simulink model "Add_1simulink"  (R2022a)
settings: Solver=FixedStepAuto  StartTime=0.0  StopTime=3  FixedStep=0.0001  RelTol=1e-3
values from neighbouring files (symbols this model uses):
  J_motor = 0.000610871894223    [var_10.mat]
  L_phase = 0.00332259990587    [var_10.mat]
  M_nom = 0.61236365542    [var_10.mat]
  psi = 0.0961787034043    [var_10.mat]
  R_phase = 0.753894801324    [var_10.mat]
  U_nom = 48    [var_10.mat]
undefined symbols (not defined in the file or in its folder): Ki_i, Ki_w, Kp_i, Kp_w
libraries: simulink x1
settings Model: Creator=Family  LastModifiedBy=Family

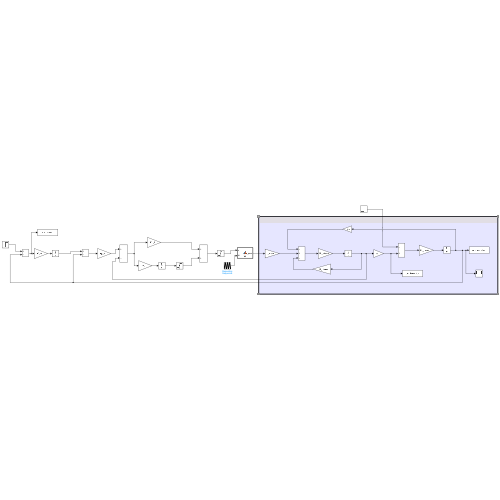
[thumbnail: Simulink's stored preview of the top-level diagram]
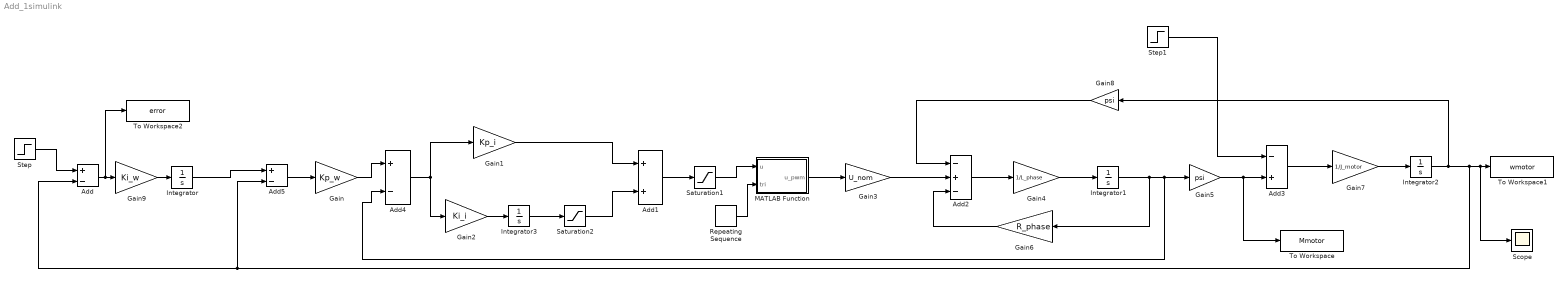
== system Add_1simulink ==
  Add : Sum  Inputs=+-
  Add1 : Sum
  Add2 : Sum  Inputs=-+-
  Add3 : Sum  Inputs=-+
  Add4 : Sum  Inputs=+-
  Add5 : Sum  Inputs=+-
  Gain : Gain  Gain=Kp_w
  Gain1 : Gain  Gain=Kp_i
  Gain2 : Gain  Gain=Ki_i
  Gain3 : Gain  Gain=U_nom
  Gain4 : Gain  Gain=1/L_phase
  Gain5 : Gain  Gain=psi
  Gain6 : Gain  Gain=R_phase
  Gain7 : Gain  Gain=1/J_motor
  Gain8 : Gain  Gain=psi
  Gain9 : Gain  Gain=Ki_w
  Integrator{,1..3} (4 alike) : Integrator
  MATLAB Function : MATLAB Function  TreatAsAtomicUnit=on
  Repeating Sequence : simulink/Sources/Repeating Sequence  rep_seq_t=[0 1/10000 1/5000]  rep_seq_y=[-1 1 -1]
  Saturation1 : Saturate  UpperLimit=1  LowerLimit=-1
  Saturation2 : Saturate  UpperLimit=1  LowerLimit=-1
  Scope : Scope
  Step : Step  Time=0.5  After=50  SampleTime=0
  Step1 : Step  Time=0.5  After=M_nom  SampleTime=0
  To Workspace : ToWorkspace  VariableName=Mmotor  SaveFormat=Timeseries  SampleTime=0.001
  To Workspace1 : ToWorkspace  VariableName=wmotor  SaveFormat=Timeseries  SampleTime=0.001
  To Workspace2 : ToWorkspace  VariableName=error  SaveFormat=Timeseries  SampleTime=0.001
  wires:
  Gain1/1 -> Add1/1
  Add1/1 -> Saturation1/1
  Gain2/1 -> Integrator3/1
  Add3/1 -> Gain7/1
  Integrator2/1 -> Add5/2, Add/2, Scope/1, To Workspace1/1, Gain8/1
  Gain7/1 -> Integrator2/1
  Gain6/1 -> Add2/3
  Gain5/1 -> To Workspace/1, Add3/2
  Gain4/1 -> Integrator1/1
  Add2/1 -> Gain4/1
  Gain3/1 -> Add2/2
  Integrator1/1 -> Gain6/1, Add4/2, Gain5/1
  Gain8/1 -> Add2/1
  Saturation1/1 -> MATLAB Function/1(u)
  Integrator3/1 -> Saturation2/1
  Saturation2/1 -> Add1/2
  Add4/1 -> Gain2/1, Gain1/1
  Gain/1 -> Add4/1
  Add/1 -> To Workspace2/1, Gain9/1
  Step/1 -> Add/1
  Gain9/1 -> Integrator/1
  Integrator/1 -> Add5/1
  MATLAB Function/1(u_pwm) -> Gain3/1
  Repeating Sequence/1 -> MATLAB Function/2(tri)
  Step1/1 -> Add3/1
  Add5/1 -> Gain/1

== matlab function Add_1simulink/MATLAB Function ==
  data: u input; u_pwm output; tri input
function u_pwm = fcn(u,tri)
if u >= tri
    u_pwm = 1;
else
    u_pwm = -1;
end
